simulink model "quart_vehicule_suspension_semi_active"  (R2018a)
settings: Solver=VariableStepAuto  StartTime=0.0  StopTime=10.0  RelTol=1e-3
settings Model: Creator=hp  LastModifiedBy=hp

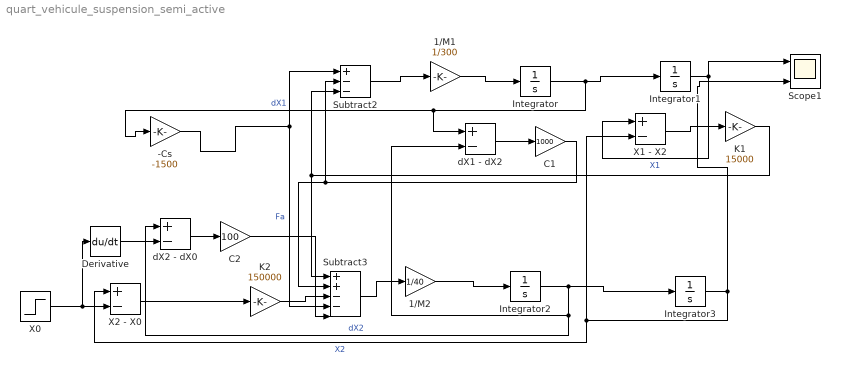
== system quart_vehicule_suspension_semi_active ==
  -Cs : Gain  Gain=-1500
  1/M1 : Gain  Gain=1/300
  1/M2 : Gain  Gain=1/40
  C1 : Gain  Gain=1000
  C2 : Gain  Gain=100
  Derivative : Derivative
  Integrator{,1..3} (4 alike) : Integrator
  K1 : Gain  Gain=15000
  K2 : Gain  Gain=150000
  Scope1 : Scope  NumInputPorts=3
  Subtract2 : Sum  Inputs=+--
  Subtract3 : Sum  Inputs=|+|+|-|-|-
  X0 : Step  After=0.05  SampleTime=0
  X1 - X2 : Sum  Inputs=+-
  X2 - X0 : Sum  Inputs=+-
  dX1 - dX2 : Sum  Inputs=+-
  dX2 - dX0 : Sum  Inputs=+-
  wires:
  Integrator/1 -> -Cs/1, dX1 - dX2/1, Integrator1/1  "dX1"
  Integrator2/1 -> dX2 - dX0/1, dX1 - dX2/2, Integrator3/1  "dX2"
  1/M1/1 -> Integrator/1
  1/M2/1 -> Integrator2/1
  Integrator1/1 -> Scope1/1, X1 - X2/1  "X1"
  dX1 - dX2/1 -> C1/1
  X1 - X2/1 -> K1/1
  Integrator3/1 -> Scope1/3, X2 - X0/1, X1 - X2/2  "X2"
  C1/1 -> Subtract3/2, Subtract2/2
  K1/1 -> Subtract3/1, Subtract2/3
  Subtract2/1 -> 1/M1/1
  Subtract3/1 -> 1/M2/1
  K2/1 -> Subtract3/3
  X0/1 -> Derivative/1, X2 - X0/2
  X2 - X0/1 -> K2/1
  -Cs/1 -> Subtract3/4, Subtract2/1  "Fa"
  dX2 - dX0/1 -> C2/1
  Derivative/1 -> dX2 - dX0/2
  C2/1 -> Subtract3/5
